simulink model "Vectorized_SampleDelay_Stream_Ex1"  (R2025a)
settings: Solver=VariableStepAuto  StartTime=0.0  StopTime=0.1  RelTol=1e-3
undefined symbols (not defined in the file): S, vsva2197, xcvc1902
libraries: dspsrcs4 x1, aieDSP x1, vmcUtilities x1
settings Model: Creator=sdegala  LastModifiedBy=robg
settings ModelReferenceCC: EnableRefExpFcnMdlSchedulingChecks=on
settings RTWCC: GPUComputeCapability=3.5

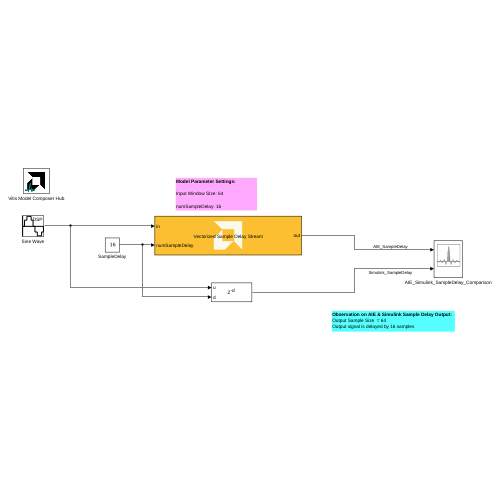
[thumbnail: Simulink's stored preview of the top-level diagram]
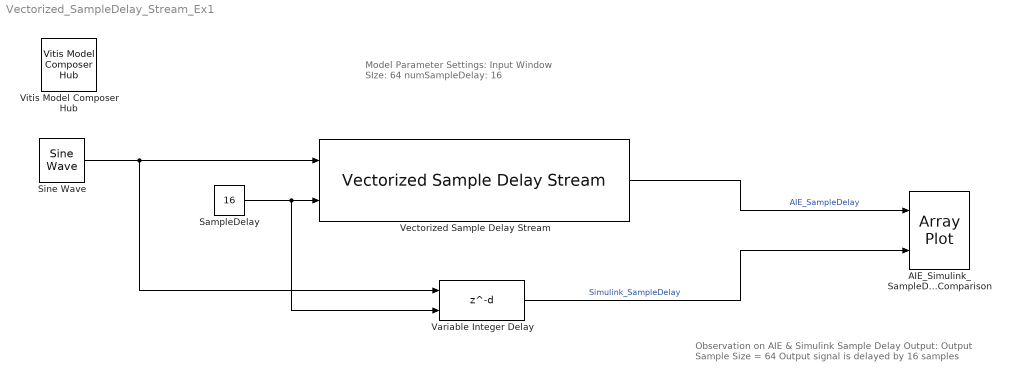
== system Vectorized_SampleDelay_Stream_Ex1 ==
  note: Observation on AIE & Simulink Sample Delay Output:
      | Output Sample Size = 64
      | Output signal is delayed by 16 samples
  note: Model Parameter Settings:
      |
      | Input Window SIze: 64
      |
      | numSampleDelay: 16
  AIE_Simulink_SampleDelay_Comparison : ArrayPlot  NumInputPorts=2  WindowPosition=[2.000000,37.000000,1280.000000,655.000000,]  PlotType=Line  YLimits=[-1.1888,1.1888]  ShowLegend=on
  SampleDelay : Constant  Value=16  OutDataTypeStr=uint32
  Sine Wave : dspsrcs4/Sine Wave  Amplitude=1  Frequency=10  Phase=0  SampleMode=Discrete  OutComplex=Real  CompMethod=Trigonometric fcn  TableSize=Speed  SampleTime=1/100  SamplesPerFrame=64  ResetState=Restart at time zero  OutputFrames=off  dataType=single  wordLen=16  udDataType=sfix(16)  fracBitsMode=Best precision  numFracBits=15  OutDataTypeStr=single  LastOutDataTypeStr=single
  Variable Integer Delay : Delay  DelayLengthSource=Input port  DelayLengthUpperLimit=256  InputProcessing=Columns as channels (frame based)
      settings: InputPortMap=u0,p1
  Vectorized Sample Delay Stream : aieDSP/Vectorized Sample Delay Stream  data_type=float  input_window_size=64  max_sample_delay=256  AIE_VARIANT=1  TP_API=0  blockJsonConstraints=[]  blockJsonConstraintsInternal=[]  spec=vmc_stream_sample_delay.json  SerializedMaskParamNames=[]  SerializedMaskParamValues=[]  SerializedMaskParamVisibilities=[]  block_type=Vectorized Sample Delay Stream  SerializedMaskParamDataypes=typename|uint|uint|uint|uint  SerializedMaskParamEnumStrArr=0|0|0|0|0  SerializedMaskParamEnumValArr=0|0|0|0|0  SerializedMaskParamVectorArr=0|0|0|0|0  SerializedMaskParamKeys=TT_DATA|TP_WINDOW_VSIZE|TP_MAX_DELAY|AIE_VARIANT|TP_API
  Vitis Model Composer Hub : vmcUtilities/Vitis Model Composer Hub  Tag=genX  CodeGeneration=off  StartColumn=1  NumberOfColumns=1  TargetDirectory=./code  exportDesign=off  analyzeDesign=off  validateDesignOnHw=off  ExportType=AI Engines  IpVendor=xilinx.com  IpLibrary=hls  IpVersion=1.0  IpHWLanguage=Verilog  AieCompilerOptions={}  AieSimulatorOptions={}  CreateTestbench=off  TestbenchStackSize=10  RunRtlSim=off  RunCSim=off  RunAieSim=off  enableSimulationTimeout=on  enableGraphIterations=on  AieSimTimeout=50000  AieGraphIterations=-1  RunAieSimProfiling=off  LaunchVitisAnalyzer=off  PlotOutput=off  RunX86Sim=off  X86SimTimeout=10  GenHwImage=off  GenLibadfXo=off  GenHwValidationCode=off  PlatformType=Not Specified  HwSystemType=Baremetal  HwValidationTarget=hw  ProjDevice=xcvc1902-vsva2197-1LP-e-S  ProjDevicePart=xcvc1902-vsva2197-1LP-e-S  AIEType=AIE  SamplePeriod=-1  ClockFrequency=200  DataPathParallelism=1  xilinxfamily=versalaicore  part=xcvc1902  speed=-1LP-e-S  package=vsva2197  directory=./netlist  testbench=off  incr_netlist=off  synthesis_tool=Vivado  clock_wrapper=Clock Enables  dbl_ovrd=According to Block Masks  dcm_input_clock_period=10  sysclk_period=10  simulink_period=1  eval_field=0  LogFileName=''  NThreads=4
  wires:
  Sine Wave/1 -> Variable Integer Delay/1, Vectorized Sample Delay Stream/1
  Variable Integer Delay/1 -> AIE_Simulink_SampleDelay_Comparison/2  "Simulink_SampleDelay"
  SampleDelay/1 -> Vectorized Sample Delay Stream/2, Variable Integer Delay/2
  Vectorized Sample Delay Stream/1 -> AIE_Simulink_SampleDelay_Comparison/1  "AIE_SampleDelay"
